simulink model "PlantModel1"  (R2022b)
settings: Solver=VariableStepAuto  StartTime=0.0  StopTime=inf  RelTol=1e-3
libraries: simulink x16, rllib x1
settings Model: Creator=Fatha  LastModifiedBy=Fatha

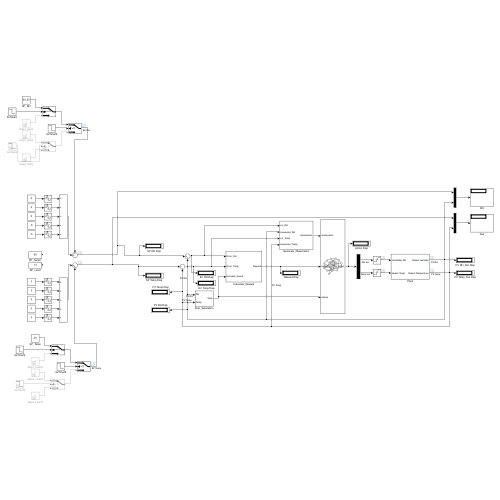
[thumbnail: Simulink's stored preview of the top-level diagram]
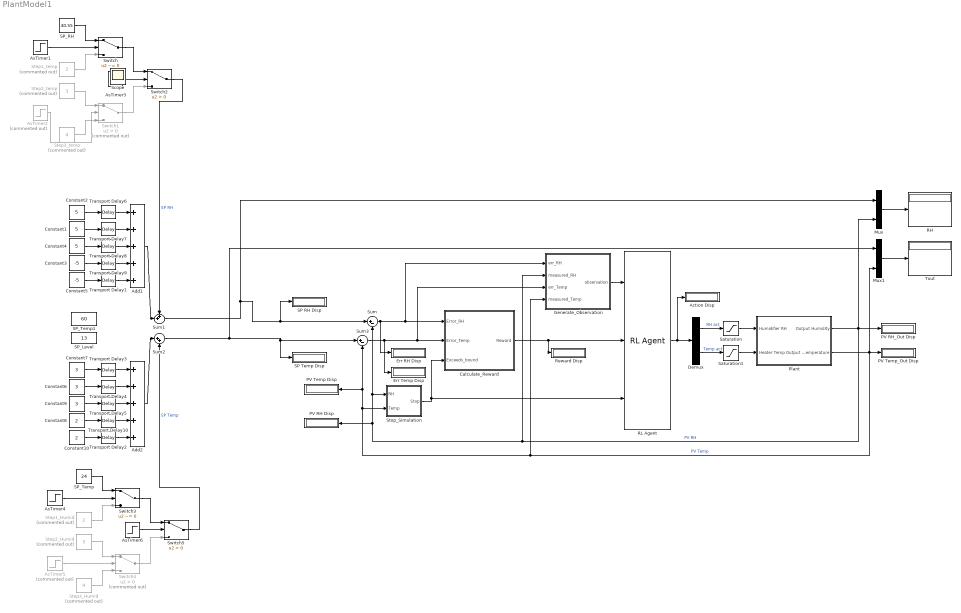
== system PlantModel1 ==
  Action Disp : Display
  Add1 : Sum  Inputs=+++++
  Add2 : Sum  Inputs=+++++
  AsTimer{1,3..4,6} (4 alike) : Step  Time=5000  Before=1  After=0  SampleTime=0
  AsTimer2 : Step  Commented=on  Time=600  Before=1  After=0  SampleTime=0
  AsTimer5 : Step  Commented=on  Time=600  Before=1  After=0  SampleTime=0
  Calculate_Reward : Subsystem
  Constant1 : Constant  Value=5
  Constant10 : Constant  Value=2
  Constant2 : Constant  Value=5
  Constant3 : Constant  Value=-5
  Constant4 : Constant  Value=5
  Constant5 : Constant  Value=-5
  Constant6 : Constant  Value=3
  Constant7 : Constant  Value=3
  Constant8 : Constant  Value=2
  Constant9 : Constant  Value=3
  Demux : Demux  Outputs=2
  Err RH Disp : Display
  Err Temp Disp : Display
  Generate_Observation : Subsystem
  Mux : Mux  Inputs=2
  Mux1 : Mux  Inputs=2
  PV RH Disp : Display
  PV RH_Out Disp : Display
  PV Temp Disp : Display
  PV Temp_Out Disp : Display
  Plant : Subsystem
  RH : Display
  RL Agent : rllib/RL Agent  Agent=agent  ExternalActionAsInput=off  ProvideLastAction=off  ProvideCumRwd=off  TreatAsDirectFeedthrough=on  UseStrictObservationDataTypes=off
  Reward Disp : Display
  SP RH Disp : Display
  SP Temp Disp : Display
  SP_Level : Constant  Value=13
  SP_RH : Constant  Value=40.55
  SP_Temp : Constant  Value=24
  SP_Temp1 : Constant  Value=60
  Saturation : Saturate  UpperLimit=100  LowerLimit=0
  Saturation1 : Saturate  UpperLimit=100  LowerLimit=0
  Step1_Humid : Constant  Commented=on  Value=2
  Step1_temp : Constant  Commented=on  Value=2
  Step2_Humid : Constant  Commented=on  Value=3
  Step2_temp : Constant  Commented=on  Value=3
  Step3_Humid : Constant  Commented=on  Value=4
  Step3_temp : Constant  Commented=on  Value=4
  Stop_Simulation : Subsystem
  Sum : Sum  Inputs=|+-
  Sum1 : Sum  Inputs=++|
  Sum2 : Sum  Inputs=|++
  Sum3 : Sum  Inputs=|+-
  Switch : Switch  Criteria=u2 ~= 0  Threshold=1  SaturateOnIntegerOverflow=off  InputSameDT=off
  Switch1 : Switch  Commented=on  Criteria=u2 > Threshold  SaturateOnIntegerOverflow=off  InputSameDT=off
  Switch2 : Switch  Criteria=u2 > Threshold  SaturateOnIntegerOverflow=off  InputSameDT=off
  Switch3 : Switch  Criteria=u2 ~= 0  Threshold=1  SaturateOnIntegerOverflow=off  InputSameDT=off
  Switch4 : Switch  Commented=on  Criteria=u2 > Threshold  SaturateOnIntegerOverflow=off  InputSameDT=off
  Switch5 : Switch  Criteria=u2 > Threshold  SaturateOnIntegerOverflow=off  InputSameDT=off
  Tout : Display
  Transport Delay1 : TransportDelay  DelayTime=3500
  Transport Delay10 : TransportDelay  DelayTime=2800
  Transport Delay2 : TransportDelay  DelayTime=3500
  Transport Delay3 : TransportDelay  DelayTime=700
  Transport Delay4 : TransportDelay  DelayTime=1400
  Transport Delay5 : TransportDelay  DelayTime=2100
  Transport Delay6 : TransportDelay  DelayTime=700
  Transport Delay7 : TransportDelay  DelayTime=1400
  Transport Delay8 : TransportDelay  DelayTime=2100
  Transport Delay9 : TransportDelay  DelayTime=2800
  Scope : Scope
  wires:
  Stop_Simulation/1(Stop) -> RL Agent/3, Calculate_Reward/3(Exceeds_bound)
  Plant/1(Output Humidity) -> Mux/2, PV RH Disp/1, Sum/2, Stop_Simulation/1(RH), Generate_Observation/2(measured_RH), PV RH_Out Disp/1  "PV RH"
  Generate_Observation/1(observation) -> RL Agent/1
  Sum3/1 -> Err Temp Disp/1, Calculate_Reward/2(Error_Temp), Generate_Observation/3(err_Temp)
  Mux1/1 -> Tout/1
  RL Agent/1 -> Demux/1, Action Disp/1
  Sum/1 -> Err RH Disp/1, Calculate_Reward/1(Error_RH), Generate_Observation/1(err_RH)
  Mux/1 -> RH/1
  Plant/2(Output Temperature) -> Stop_Simulation/2(Temp), PV Temp Disp/1, Sum3/2, Generate_Observation/4(measured_Temp), PV Temp_Out Disp/1, Mux1/2  "PV Temp"
  Calculate_Reward/1(Reward) -> Reward Disp/1, RL Agent/2
  Demux/1 -> Saturation/1  "RH act"
  Demux/2 -> Saturation1/1  "Temp act"
  Saturation/1 -> Plant/1(Humidifier RH)
  Saturation1/1 -> Plant/2(Heater Temp)
  AsTimer3/1 -> Switch2/2
  AsTimer2/1 -> Switch1/2
  Step3_temp/1 -> Switch1/3
  AsTimer1/1 -> Switch/2
  Step2_temp/1 -> Switch1/1
  Switch1/1 -> Switch2/3
  Step1_temp/1 -> Switch/3
  SP_RH/1 -> Switch/1
  Switch/1 -> Switch2/1
  SP_Temp/1 -> Switch3/1
  Switch4/1 -> Switch5/3
  Switch3/1 -> Switch5/1
  AsTimer4/1 -> Switch3/2
  Step1_Humid/1 -> Switch3/3
  Step3_Humid/1 -> Switch4/3
  AsTimer5/1 -> Switch4/2
  AsTimer6/1 -> Switch5/2
  Step2_Humid/1 -> Switch4/1
  Sum1/1 -> Mux/1, Sum/1, SP RH Disp/1
  Sum2/1 -> SP Temp Disp/1, Sum3/1, Mux1/1
  Transport Delay6/1 -> Add1/1
  Constant4/1 -> Transport Delay8/1
  Transport Delay1/1 -> Add1/5
  Constant10/1 -> Transport Delay2/1
  Constant6/1 -> Transport Delay4/1
  Transport Delay4/1 -> Add2/2
  Transport Delay9/1 -> Add1/4
  Constant2/1 -> Transport Delay6/1
  Transport Delay3/1 -> Add2/1
  Constant7/1 -> Transport Delay3/1
  Transport Delay2/1 -> Add2/5
  Constant3/1 -> Transport Delay9/1
  Transport Delay5/1 -> Add2/3
  Constant9/1 -> Transport Delay5/1
  Transport Delay10/1 -> Add2/4
  Transport Delay7/1 -> Add1/2
  Constant1/1 -> Transport Delay7/1
  Constant8/1 -> Transport Delay10/1
  Transport Delay8/1 -> Add1/3
  Constant5/1 -> Transport Delay1/1
  Switch2/1 -> Sum1/1  "SP RH"
  Switch5/1 -> Sum2/2  "SP Temp"
  Add2/1 -> Sum2/1
  Add1/1 -> Sum1/2

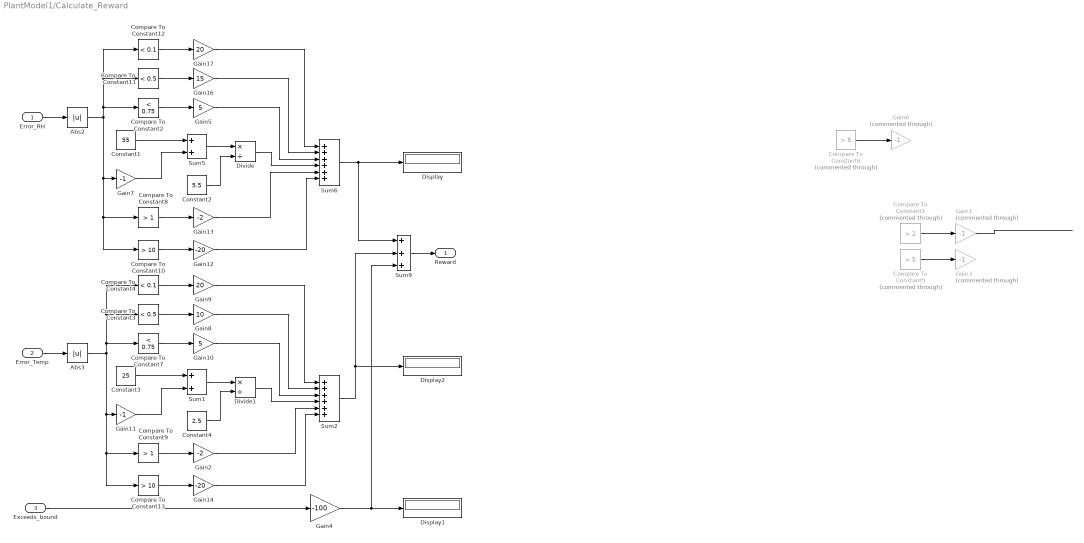
== system PlantModel1/Calculate_Reward ==
  Error_RH : Inport
  Error_Temp : Inport  Port=2
  Exceeds_bound : Inport  Port=3
  Abs2 : Abs  SaturateOnIntegerOverflow=off
  Abs3 : Abs  SaturateOnIntegerOverflow=off
  Compare To Constant1 : simulink/Logic and Bit Operations/Compare To Constant  Commented=through  relop=>  const=2  OutDataTypeStr=boolean
  Compare To Constant10 : simulink/Logic and Bit Operations/Compare To Constant  relop=>  const=10  OutDataTypeStr=boolean
  Compare To Constant11 : simulink/Logic and Bit Operations/Compare To Constant  relop=<  const=0.5  OutDataTypeStr=boolean
  Compare To Constant12 : simulink/Logic and Bit Operations/Compare To Constant  relop=<  const=0.1  OutDataTypeStr=boolean
  Compare To Constant13 : simulink/Logic and Bit Operations/Compare To Constant  relop=>  const=10  OutDataTypeStr=boolean
  Compare To Constant2 : simulink/Logic and Bit Operations/Compare To Constant  relop=<  const=0.75  OutDataTypeStr=boolean
  Compare To Constant3 : simulink/Logic and Bit Operations/Compare To Constant  relop=<  const=0.5  OutDataTypeStr=boolean
  Compare To Constant4 : simulink/Logic and Bit Operations/Compare To Constant  relop=<  const=0.1  OutDataTypeStr=boolean
  Compare To Constant5 : simulink/Logic and Bit Operations/Compare To Constant  Commented=through  relop=>  const=5  OutDataTypeStr=boolean
  Compare To Constant6 : simulink/Logic and Bit Operations/Compare To Constant  Commented=through  relop=>  const=5  OutDataTypeStr=boolean
  Compare To Constant7 : simulink/Logic and Bit Operations/Compare To Constant  relop=<  const=0.75  OutDataTypeStr=boolean
  Compare To Constant8 : simulink/Logic and Bit Operations/Compare To Constant  relop=>  const=1  OutDataTypeStr=boolean
  Compare To Constant9 : simulink/Logic and Bit Operations/Compare To Constant  relop=>  const=1  OutDataTypeStr=boolean
  Constant1 : Constant  Value=55
  Constant2 : Constant  Value=5.5
  Constant3 : Constant  Value=25
  Constant4 : Constant  Value=2.5
  Display : Display
  Display1 : Display
  Display2 : Display
  Divide : Product  Inputs=*/
  Divide1 : Product  Inputs=*/
  Gain1 : Gain  Commented=through  Gain=-1
  Gain10 : Gain  Gain=5
  Gain11 : Gain  Gain=-1
  Gain12 : Gain  Gain=-20
  Gain13 : Gain  Gain=-2
  Gain14 : Gain  Gain=-20
  Gain16 : Gain  Gain=15
  Gain17 : Gain  Gain=20
  Gain2 : Gain  Gain=-2
  Gain3 : Gain  Commented=through  Gain=-1
  Gain4 : Gain  Gain=-100
  Gain5 : Gain  Gain=5
  Gain6 : Gain  Commented=through  Gain=-1
  Gain7 : Gain  Gain=-1
  Gain8 : Gain  Gain=10
  Gain9 : Gain  Gain=20
  Sum1 : Sum
  Sum2 : Sum  Inputs=6
  Sum5 : Sum
  Sum6 : Sum  Inputs=6
  Sum9 : Sum  Inputs=+++
  Reward : Outport
  wires:
  Compare To Constant2/1 -> Gain5/1
  Constant1/1 -> Sum5/1
  Gain7/1 -> Sum5/2
  Gain5/1 -> Sum6/3
  Sum5/1 -> Divide/1
  Constant2/1 -> Divide/2
  Abs2/1 -> Compare To Constant2/1, Compare To Constant11/1, Compare To Constant12/1, Compare To Constant10/1, Compare To Constant8/1, Gain7/1
  Error_Temp/1 -> Abs3/1
  Error_RH/1 -> Abs2/1
  Exceeds_bound/1 -> Gain4/1
  Sum6/1 -> Sum9/1, Display/1
  Gain4/1 -> Display1/1, Sum9/3
  Sum9/1 -> Reward/1
  Compare To Constant6/1 -> Gain6/1
  Compare To Constant5/1 -> Gain3/1
  Compare To Constant1/1 -> Gain1/1
  Gain1/1 -> ?
  ? -> Compare To Constant1/1
  Compare To Constant8/1 -> Gain13/1
  Compare To Constant11/1 -> Gain16/1
  Gain16/1 -> Sum6/2
  Compare To Constant12/1 -> Gain17/1
  Gain17/1 -> Sum6/1
  Divide/1 -> Sum6/4
  Gain13/1 -> Sum6/5
  Gain2/1 -> Sum2/5
  Divide1/1 -> Sum2/4
  Gain9/1 -> Sum2/1
  Compare To Constant4/1 -> Gain9/1
  Gain8/1 -> Sum2/2
  Compare To Constant3/1 -> Gain8/1
  Compare To Constant9/1 -> Gain2/1
  Abs3/1 -> Gain11/1, Compare To Constant13/1, Compare To Constant9/1, Compare To Constant4/1, Compare To Constant3/1, Compare To Constant7/1
  Constant4/1 -> Divide1/2
  Sum1/1 -> Divide1/1
  Gain10/1 -> Sum2/3
  Gain11/1 -> Sum1/2
  Constant3/1 -> Sum1/1
  Compare To Constant7/1 -> Gain10/1
  Sum2/1 -> Display2/1, Sum9/2
  Compare To Constant10/1 -> Gain12/1
  Gain12/1 -> Sum6/6
  Compare To Constant13/1 -> Gain14/1
  Gain14/1 -> Sum2/6

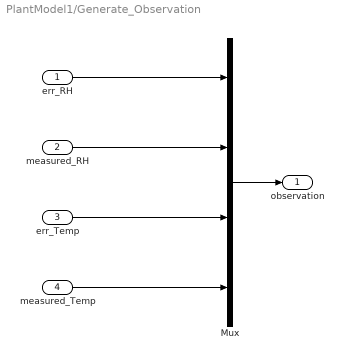
== system PlantModel1/Generate_Observation ==
  err_RH : Inport
  measured_RH : Inport  Port=2
  err_Temp : Inport  Port=3
  measured_Temp : Inport  Port=4
  Mux : Mux
  observation : Outport
  wires:
  Mux/1 -> observation/1
  err_RH/1 -> Mux/1
  measured_RH/1 -> Mux/2
  err_Temp/1 -> Mux/3
  measured_Temp/1 -> Mux/4

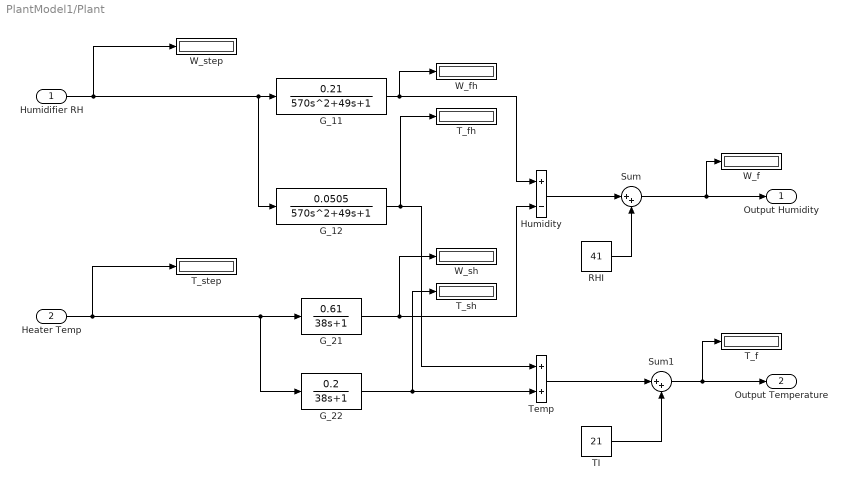
== system PlantModel1/Plant ==
  Humidifier RH : Inport
  Heater Temp : Inport  Port=2
  G_11 : TransferFcn  Numerator=[0.21]  Denominator=[570 49 1]
  G_12 : TransferFcn  Numerator=[0.0505]  Denominator=[570 49 1]
  G_21 : TransferFcn  Numerator=[0.61]  Denominator=[38 1]
  G_22 : TransferFcn  Numerator=[0.2]  Denominator=[38 1]
  Humidity : Sum  Inputs=+-
  RHI : Constant  Value=41
  Sum : Sum  Inputs=|++
  Sum1 : Sum  Inputs=|++
  TI : Constant  Value=21
  T_f : Display
      settings: Decimation=6
  T_fh : Display
      settings: Decimation=6
  T_sh : Display
      settings: Decimation=6
  T_step : Display
      settings: Decimation=6
  Temp : Sum
  W_f : Display
      settings: Decimation=6
  W_fh : Display
      settings: Decimation=6
  W_sh : Display
      settings: Decimation=6
  W_step : Display
      settings: Decimation=6
  Output Humidity : Outport
  Output Temperature : Outport  Port=2
  wires:
  G_21/1 -> W_sh/1, Humidity/2
  G_12/1 -> T_fh/1, Temp/1
  G_22/1 -> T_sh/1, Temp/2
  G_11/1 -> W_fh/1, Humidity/1
  Humidity/1 -> Sum/1
  Sum/1 -> W_f/1, Output Humidity/1
  Sum1/1 -> T_f/1, Output Temperature/1
  Temp/1 -> Sum1/1
  Heater Temp/1 -> G_22/1, G_21/1, T_step/1
  Humidifier RH/1 -> G_12/1, G_11/1, W_step/1
  RHI/1 -> Sum/2
  TI/1 -> Sum1/2

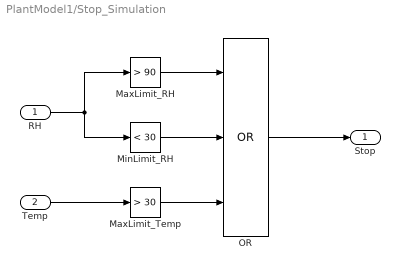
== system PlantModel1/Stop_Simulation ==
  RH : Inport
  Temp : Inport  Port=2
  MaxLimit_RH : simulink/Logic and Bit Operations/Compare To Constant  relop=>  const=90  OutDataTypeStr=boolean
  MaxLimit_Temp : simulink/Logic and Bit Operations/Compare To Constant  relop=>  const=30  OutDataTypeStr=boolean
  MinLimit_RH : simulink/Logic and Bit Operations/Compare To Constant  relop=<  const=30  OutDataTypeStr=boolean
  OR : Logic  Operator=OR  Inputs=3  IconShape=distinctive  AllPortsSameDT=off  OutDataTypeStr=boolean
  Stop : Outport
  wires:
  Temp/1 -> MaxLimit_Temp/1
  MinLimit_RH/1 -> OR/2
  RH/1 -> MinLimit_RH/1, MaxLimit_RH/1
  MaxLimit_RH/1 -> OR/1
  MaxLimit_Temp/1 -> OR/3
  OR/1 -> Stop/1
